simulink model "problem4"  (R2020b)
settings: Solver=VariableStepAuto  StartTime=0.0  StopTime=10.0  RelTol=1e-3
undefined symbols (not defined in the file): b, J, K, L, R
settings Model: Creator=Shivashis  LastModifiedBy=Shivashis

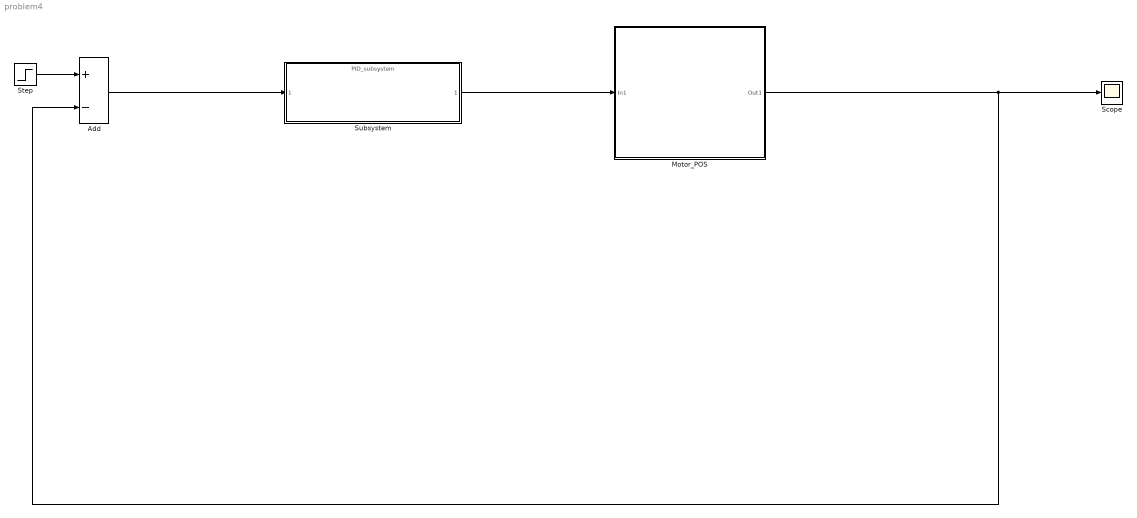
== system problem4 ==
  Add : Sum  Inputs=+-
  Motor_POS : Subsystem
  Scope : Scope
  Step : Step  SampleTime=0
  Subsystem : ModelReference  ModelNameDialog=PID_subsystem  SimulationMode=Normal  ModelReferenceVersion=1.6
  wires:
  Step/1 -> Add/1
  Add/1 -> Subsystem/1
  Motor_POS/1(Out1) -> Add/2, Scope/1
  Subsystem/1 -> Motor_POS/1(In1)

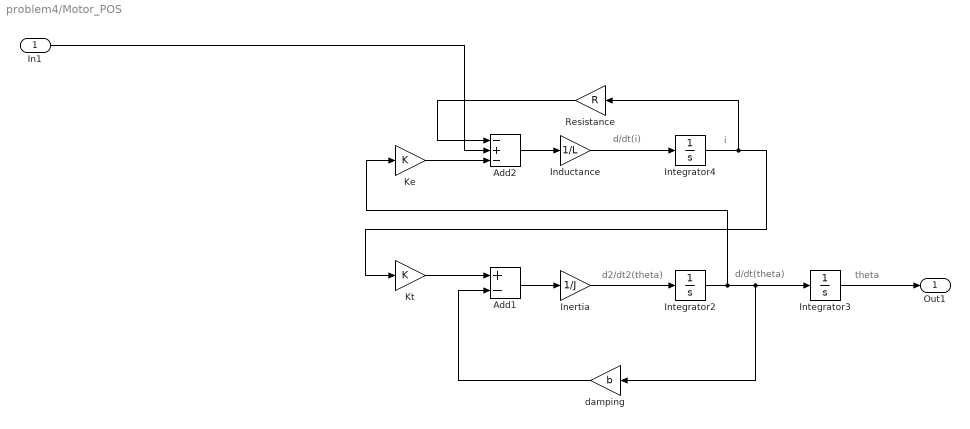
== system problem4/Motor_POS ==
  note: i
  note: d2/dt2(theta)
  note: d/dt(theta)
  note: theta
  note: d/dt(i)
  In1 : Inport
  Add1 : Sum  Inputs=+-
  Add2 : Sum  Inputs=-+-
  Inductance : Gain  Gain=1/L
  Inertia : Gain  Gain=1/J
  Integrator2 : Integrator
  Integrator3 : Integrator
  Integrator4 : Integrator
  Ke : Gain  Gain=K
  Kt : Gain  Gain=K
  Resistance : Gain  Gain=R
  damping : Gain  Gain=b
  Out1 : Outport
  wires:
  Resistance/1 -> Add2/1
  Integrator2/1 -> Ke/1, damping/1, Integrator3/1
  Add1/1 -> Inertia/1
  Integrator4/1 -> Resistance/1, Kt/1
  Inertia/1 -> Integrator2/1
  Add2/1 -> Inductance/1
  damping/1 -> Add1/2
  Kt/1 -> Add1/1
  Ke/1 -> Add2/3
  Inductance/1 -> Integrator4/1
  In1/1 -> Add2/2
  Integrator3/1 -> Out1/1
